simulink model "part_3_linear"  (R2018b)
settings: Solver=VariableStepAuto  StartTime=0.0  StopTime=t_f  RelTol=1e-3
values from neighbouring files (symbols this model uses):
  alpha_final = 3*pi/180    (= 0.0523598775598)    [Part_3.m]
  alpha_initial = 0    [Part_3.m]
  alpha_step_time = 15    [Part_3.m]
  G1 = tf(zpk([-0.065],[-0.013],[41]))    [Part_3.m]
  G_2_1 = tf(G_2_1)    [Part_3.m]
  G_2_2 = tf(G_2_2)    [Part_3.m]
  v_final = 31.2928    [Part_3.m]
  v_initial = 26.8224    [Part_3.m]
  v_step_time = 1    [Part_3.m]
settings Model: Creator=Nick Carcione  LastModifiedBy=Nick Carcione

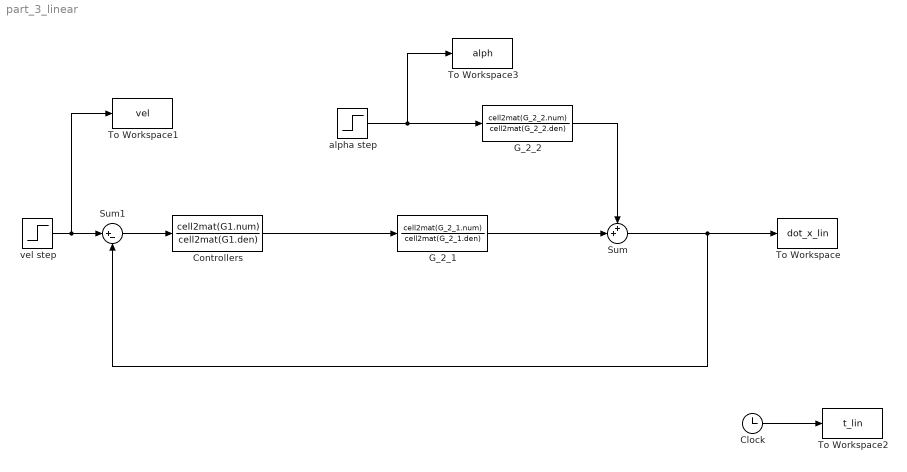
== system part_3_linear ==
  Clock : Clock
  Controllers : TransferFcn  Numerator=cell2mat(G1.num)  Denominator=cell2mat(G1.den)
  G_2_1 : TransferFcn  Numerator=cell2mat(G_2_1.num)  Denominator=cell2mat(G_2_1.den)
  G_2_2 : TransferFcn  Numerator=cell2mat(G_2_2.num)  Denominator=cell2mat(G_2_2.den)
  Sum : Sum  Inputs=++|
  Sum1 : Sum  Inputs=|+-
  To Workspace : ToWorkspace  VariableName=dot_x_lin  SampleTime=-1
  To Workspace1 : ToWorkspace  VariableName=vel  SampleTime=-1
  To Workspace2 : ToWorkspace  VariableName=t_lin  SampleTime=-1
  To Workspace3 : ToWorkspace  VariableName=alph  SampleTime=-1
  alpha step : Step  Time=alpha_step_time  Before=alpha_initial  After=alpha_final  SampleTime=0
  "vel step " : Step  Time=v_step_time  Before=v_initial  After=v_final  SampleTime=0
  wires:
  Controllers/1 -> G_2_1/1
  G_2_1/1 -> Sum/2
  G_2_2/1 -> Sum/1
  alpha step/1 -> To Workspace3/1, G_2_2/1
  "vel step "/1 -> To Workspace1/1, Sum1/1
  Sum1/1 -> Controllers/1
  Sum/1 -> Sum1/2, To Workspace/1
  Clock/1 -> To Workspace2/1
